simulink model "Capstone_Prooject"  (R2022b)
settings: Solver=VariableStepAuto  StartTime=0.0  StopTime=10  RelTol=1e-3
libraries: simulink_extras x7, vehdynlibsteering x1, autolibshared x1
settings Model: Creator=Lenovo  LastModifiedBy=ASUS

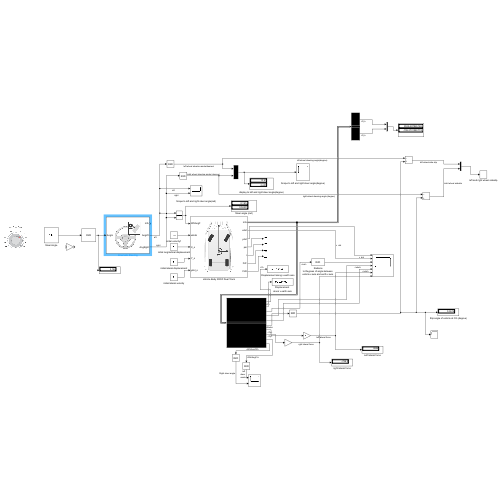
[thumbnail: Simulink's stored preview of the top-level diagram]
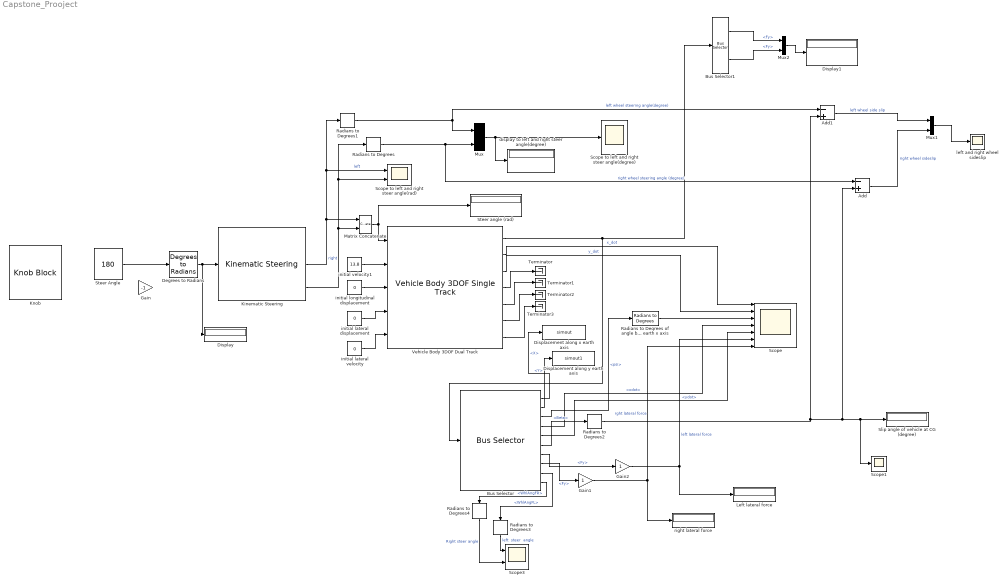
== system Capstone_Prooject ==
  " Scope to left and right steer angle(rad)" : Scope  NumInputPorts=2
  Add : Sum  Inputs=-+
  Add1 : Sum  Inputs=-+
  Bus Selector : BusSelector  OutputSignals=InertFrm.Cg.Disp.X,InertFrm.Cg.Disp.Y,InertFrm.Cg.Ang.psi,BdyFrm.Cg.Vel.xdot,BdyFrm.Cg.Vel.ydot,BdyFrm.Cg.Ang.Beta,BdyFrm.Forces.FrntAxl.Lft.Fy,BdyFrm.Forces.FrntAxl.Rght.Fy,BdyFrm.FrntAxl.Steer.WhlAngFL,BdyFrm.FrntAxl.Steer.WhlAngFR
  Bus Selector1 : BusSelector  OutputSignals=BdyFrm.Forces.Tires.FrntTires.Lft.Fy,BdyFrm.Forces.Tires.FrntTires.Rght.Fy
  Degrees to Radians : simulink_extras/Transformations/Degrees to Radians
  Displacement along y earth axis : ToWorkspace  VariableName=simout1  SampleTime=-1
      settings: Save2DSignal=2-D array (concatenate along first dimension)
  Displacement along x earth axis : ToWorkspace  VariableName=simout  SampleTime=-1
      settings: Save2DSignal=2-D array (concatenate along first dimension)
  Display : Display
  Display1 : Display
  Gain : Gain  Gain=-1
  Gain1 : Gain
  Gain2 : Gain
  Kinematic Steering : vehdynlibsteering/Kinematic Steering  StrgType=Rack and pinion  StrgRatioType=Constant  Loc=Front  NrmlFctr=0.01  TrckWdth=1.475  WhlBase=1.524  Db=0  StrgRng=6*pi  StrgAngBpts="[-6.2832   -5.0265   -3.7699   -2.5133   -1.2566         0    1.2566    2.5133    3.7699    5.0265    6.2832]"  StrgRatioTbl=|  StrgRatio=100  PctAckIn=off  PctAck=100  PctAckTbl=ones(1,11)*100  StrgArmLngth=0.3  RckCsLngth=0.65  TieRodLngth=0.13  D=0.12  PnnRadius=0.007  PnnRadiusTbl="[0.0055    0.0055    0.0056    0.0057    0.0058    0.0057    0.0057    0.0057    0.0056    0.0055    0.0055]"  RodLngth=0.1  ParaArmLngth=0.9  aMode=2
      | [13.5000   13.3750   13.2500   13.1250   13.0000   13.0000   13.0000   13.1250   13.2500   13.3750   13.5000
      | ]
  Knob : KnobBlock  ScaleMin=-540  ScaleMax=540
  Left lateral force : Display
  Matrix Concatenate : Concatenate  ConcatenateDimension=2
  Mux : Mux  Inputs=2
  Mux1 : Mux  Inputs=2
  Mux2 : Mux  Inputs=2
  Radians to Degrees{,1..4} (5 alike) : simulink_extras/Transformations/Radians to Degrees
  "Radians to Degrees of angle between vehicle x axis and earth x axis " : simulink_extras/Transformations/Radians to Degrees
  Scope : Scope  NumInputPorts=7
  Scope to left and right steer angle(degree) : Scope
  Scope1 : Scope
  Scope3 : Scope  NumInputPorts=2
  Slip angle of vehicle at CG (degree) : Display
  Steer Angle : Constant  Value=180
  Steer angle (rad) : Display
  Terminator{,1..3} (4 alike) : Terminator
  Vehicle Body 3DOF Dual Track : autolibshared/Vehicle Body 3DOF Single Track  trackMode=Dual  inputMode=External longitudinal velocity  frontSteerMode=on  rearSteerMode=off  windMode=off  muMode=off  extFMode=off  extMMode=off  htchFMode=off  htchMMode=off  extXo=on  extpsio=off  extxdoto=off  extro=off  extYo=on  extTamb=off  extydoto=on  aMode=2  NF=2  NR=2  m=2000  a=1.4  b=1.6  h=0.35  dh=1  hh=0.2  X_o=0  xdot_o=0  CalphaMode=off  sigmaMode=on  d=0  hl=0  w=[1.4,1.4]  Cy_f=52000  Cy_r=64000  sigma_f=.1  sigma_r=.1  alpha_f_brk=[-.1 .1]  Cy_f_data=[-9e3 9e3]  alpha_r_brk=[-.1 .1]  Cy_r_data=[-9e3 9e3]  Y_o=0  ydot_o=0  Izz=3600  psi_o=0  r_o=0  Af=2  Cd=.3  Cl=.1  Cpm=.1  beta_w=[0 0.01:0.01:0.3]  Cs=[0:0.03:0.9]  Cym=[0 1e-6:0.01:0.3]  Pabs=101325  Tair=273  g=9.81  mu=1  xdot_tol=.01  Fznom=5000  Fxtire_sat=7e4  Fytire_sat=7e4  longOff=0  latOff=0  vertOff=0  wrapAng=off
      settings: LibrarySourceBlock=vehdynlibeom/Vehicle Body 3DOF Dual Track
  display to left and right steer angle(degree) : Display
  initial lateral displacement : Constant  Value=0
  initial lateral velocity : Constant  Value=0
  initial longitudinal displacement : Constant  Value=0
  initial velocity1 : Constant  Value=13.8
  left and right wheel sideslip : Scope
  right lateral force : Display
  wires:
  Kinematic Steering/3 -> Radians to Degrees/1, " Scope to left and right steer angle(rad)"/2, Matrix Concatenate/2  "right"
  Kinematic Steering/2 -> Radians to Degrees1/1, " Scope to left and right steer angle(rad)"/1, Matrix Concatenate/1  "left"
  Matrix Concatenate/1 -> Vehicle Body 3DOF Dual Track/1, Steer angle (rad)/1
  Vehicle Body 3DOF Dual Track/2 -> Scope/1  "x_dot"
  Vehicle Body 3DOF Dual Track/3 -> Scope/2  "y_dot"
  Vehicle Body 3DOF Dual Track/1 -> Bus Selector1/1, Bus Selector/1
  Bus Selector/3 -> "Radians to Degrees of angle between vehicle x axis and earth x axis "/1  "<psi>"
  Bus Selector/4 -> Scope/4  "<xdot>"
  Bus Selector/5 -> Scope/5  "<ydot>"
  Radians to Degrees/1 -> Add/1, Mux/2  "right wheel steering angle (degree)"
  Radians to Degrees1/1 -> Add1/1, Mux/1  "left wheel steering angle(degree)"
  initial longitudinal displacement/1 -> Vehicle Body 3DOF Dual Track/3
  initial lateral displacement/1 -> Vehicle Body 3DOF Dual Track/4
  Bus Selector/1 -> Displacement along x earth axis/1  "<X>"
  Bus Selector/2 -> Displacement along y earth axis/1  "<Y>"
  Steer Angle/1 -> Degrees to Radians/1
  Bus Selector/6 -> Radians to Degrees2/1  "<Beta>"
  Vehicle Body 3DOF Dual Track/4 -> Terminator/1
  Vehicle Body 3DOF Dual Track/5 -> Terminator1/1
  Vehicle Body 3DOF Dual Track/6 -> Terminator2/1
  Vehicle Body 3DOF Dual Track/7 -> Terminator3/1
  Mux/1 -> display to left and right steer angle(degree)/1, Scope to left and right steer angle(degree)/1
  "Radians to Degrees of angle between vehicle x axis and earth x axis "/1 -> Scope/3
  Radians to Degrees2/1 -> Add1/2, Add/2, Scope1/1, Slip angle of vehicle at CG (degree)/1
  Add1/1 -> Mux1/1  "left wheel side slip"
  Add/1 -> Mux1/2  "right wheel sideslip"
  Mux1/1 -> left and right wheel sideslip/1
  initial lateral velocity/1 -> Vehicle Body 3DOF Dual Track/5
  initial velocity1/1 -> Vehicle Body 3DOF Dual Track/2
  Bus Selector/8 -> Gain1/1  "<Fy>"
  Bus Selector/7 -> Gain2/1  "<Fy>"
  Gain2/1 -> Left lateral force/1, Scope/6  "left lateral force"
  Gain1/1 -> Scope/7, right lateral force/1  "rght lateral force"
  Degrees to Radians/1 -> Display/1, Kinematic Steering/1
  Bus Selector/9 -> Radians to Degrees3/1  "<WhlAngFL>"
  Bus Selector/10 -> Radians to Degrees4/1  "<WhlAngFR>"
  Radians to Degrees3/1 -> Scope3/1  "left  steer  angle"
  Radians to Degrees4/1 -> Scope3/2  "Right steer angle"
  Bus Selector1/1 -> Mux2/1  "<Fy>"
  Bus Selector1/2 -> Mux2/2  "<Fy>"
  Mux2/1 -> Display1/1
